simulink model "ilk_dosya"  (R2018a)
settings: Solver=VariableStepAuto  StartTime=0.0  StopTime=10.0  RelTol=1e-3
settings Model: Creator=PC_393_ADMIN  LastModifiedBy=PC_393_ADMIN

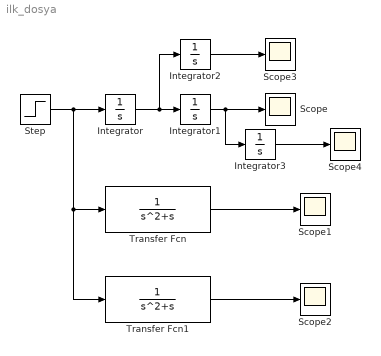
== system ilk_dosya ==
  Integrator{,1..3} (4 alike) : Integrator
  Scope{,1..4} (5 alike) : Scope
  Step : Step  SampleTime=0
  Transfer Fcn : TransferFcn  Denominator=[1 1 0]
  Transfer Fcn1 : TransferFcn  Denominator=[1 1 0]
  wires:
  Step/1 -> Transfer Fcn1/1, Transfer Fcn/1, Integrator/1
  Integrator1/1 -> Integrator3/1, Scope/1
  Transfer Fcn/1 -> Scope1/1
  Transfer Fcn1/1 -> Scope2/1
  Integrator2/1 -> Scope3/1
  Integrator/1 -> Integrator2/1, Integrator1/1
  Integrator3/1 -> Scope4/1
